simulink library "DiSC_ToolboxOpal_V12"  (R2012b)
settings: Solver=ode45  StartTime=0.0  StopTime=10.0  RelTol=1e-3
undefined symbols (not defined in the file or in its folder): SamplingTime
(part 2 of 5)

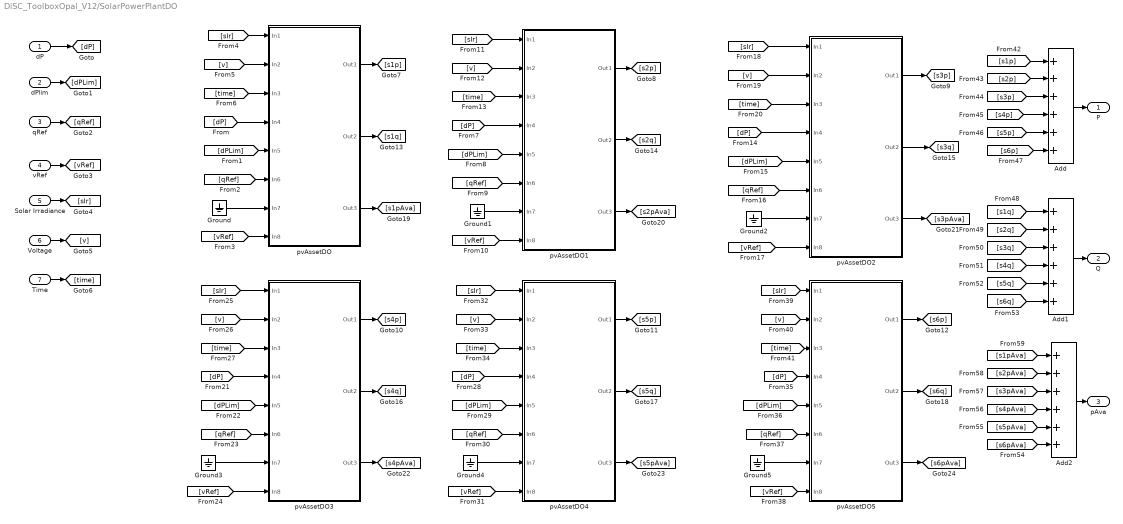
== system DiSC_ToolboxOpal_V12/SolarPowerPlantDO ==
  dP : Inport
  dPlim : Inport  Port=2
  qRef : Inport  Port=3
  vRef : Inport  Port=4
  Solar Irradiance : Inport  Port=5
  Voltage : Inport  Port=6
  Time : Inport  Port=7
  Add : Sum  Inputs=++++++
  Add1 : Sum  Inputs=++++++
  Add2 : Sum  Inputs=++++++
  Ground{,1..5} (6 alike) : Ground
  pvAssetDO : Subsystem
      mask help:
      | %pvAssetDO implements a simple P,Q controllable solar PV system using MATLAB embedded function.
      |     %   The pvAsset can be set to follow an active power reference, output
      |     %   maximum power available or derate power. It can also, at the same
      |     %   time be set to follow a reactive power reference, output the
      |     %   minimum reactive power according to the power factor or try to keep
      |     %   a voltage reference in the coupling point by controlling reactive
      |     %   power output.
      |     %
      |     %
      |     % Revision:
      |     % 19-06-2014, R. Pedersen, Aalborg University. Notes:
      |     % R. Pedersen 11-6-2014, Aalborg University
      |     % 29-11-2014, R. Olsen/M. Kemal, Aalborg University (Simulink)
      |     % 20-06-2015, F. Iov/M. Kemal, Aalborg University (Simulink toolbox for OPAL)
      |
      |                 % Input:
      |             %   - s [w/m^2], is the solar irradiance.
      |             %   - v [V], is the voltage at the connection point.
      |             %   - dP [PU], is the reference to active power change (curtailment).
      |             %   - dPlim [PU], is the reference to derated power (derate)
      |             %   - qRef [VAR], is the reactive power reference.
      |             %   - vRef [V], is the voltage reference.
      |             %
      |             % Output:
      |             %   - p [W], is the active power output
      |             %   - q [VAR], is the reactive power output
      |             %   - pAva [W], is the available power
      mask Help:
      | %pvAssetDO implements a simple P,Q controllable solar PV system using MATLAB embedded function.
      |     %   The pvAsset can be set to follow an active power reference, output
      |     %   maximum power available or derate power. It can also, at the same
      |     %   time be set to follow a reactive power reference, output the
      |     %   minimum reactive power according to the power factor or try to keep
      |     %   a voltage reference in the coupling point by controlling reactive
      |     %   power output.
      |     %
      |     %
      |     % Revision:
      |     % 19-06-2014, R. Pedersen, Aalborg University. Notes:
      |     % R. Pedersen 11-6-2014, Aalborg University
      |     % 29-11-2014, R. Olsen/M. Kemal, Aalborg University (Simulink)
      |     % 20-06-2015, F. Iov/M. Kemal, Aalborg University (Simulink toolbox for OPAL)
      | 
      |                 % Input:
      |             %   - s [w/m^2], is the solar irradiance.
      |             %   - v [V], is the voltage at the connection point.
      |             %   - dP [W], is the reference to active power change.
      |             %   - dPlim [W], is the reference to derated power.
      |             %   - qRef [VAR], is the reactive power reference.
      |             %   - vRef [V], is the voltage reference.
      |             %
      |             % Output:
      |             %   - p [W], is the active power output
      |             %   - q [VAR], is the reactive power output
      |             %   - pAva [W], is the available power
      mask Display:
      | %image(imread( 'PhotoVoltaic.png'))
      | port_label( 'output',1, 'p')
      | port_label( 'output',2, 'q')
      | port_label( 'output',3, 'pAva')
      | 
      | 
      | port_label( 'input',1, 'solarIrr')
      | port_label( 'input',2, 'vMeas')
      | port_label( 'input',3, 'time')
      | port_label( 'input',4, 'dp')
      | port_label( 'input',5, 'dplim')
      | port_label( 'input',6, 'qRef')
      | port_label( 'input',7, 'qMode')
      | port_label( 'input',8, 'vRef')
  pvAssetDO1 : Subsystem
      mask help:
      | %pvAssetDO implements a simple P,Q controllable solar PV system using MATLAB embedded function.
      |     %   The pvAsset can be set to follow an active power reference, output
      |     %   maximum power available or derate power. It can also, at the same
      |     %   time be set to follow a reactive power reference, output the
      |     %   minimum reactive power according to the power factor or try to keep
      |     %   a voltage reference in the coupling point by controlling reactive
      |     %   power output.
      |     %
      |     %
      |     % Revision:
      |     % 19-06-2014, R. Pedersen, Aalborg University. Notes:
      |     % R. Pedersen 11-6-2014, Aalborg University
      |     % 29-11-2014, R. Olsen/M. Kemal, Aalborg University (Simulink)
      |     % 20-06-2015, F. Iov/M. Kemal, Aalborg University (Simulink toolbox for OPAL)
      |
      |                 % Input:
      |             %   - s [w/m^2], is the solar irradiance.
      |             %   - v [V], is the voltage at the connection point.
      |             %   - dP [PU], is the reference to active power change (curtailment).
      |             %   - dPlim [PU], is the reference to derated power (derate)
      |             %   - qRef [VAR], is the reactive power reference.
      |             %   - vRef [V], is the voltage reference.
      |             %
      |             % Output:
      |             %   - p [W], is the active power output
      |             %   - q [VAR], is the reactive power output
      |             %   - pAva [W], is the available power
      mask Help:
      | %pvAssetDO implements a simple P,Q controllable solar PV system using MATLAB embedded function.
      |     %   The pvAsset can be set to follow an active power reference, output
      |     %   maximum power available or derate power. It can also, at the same
      |     %   time be set to follow a reactive power reference, output the
      |     %   minimum reactive power according to the power factor or try to keep
      |     %   a voltage reference in the coupling point by controlling reactive
      |     %   power output.
      |     %
      |     %
      |     % Revision:
      |     % 19-06-2014, R. Pedersen, Aalborg University. Notes:
      |     % R. Pedersen 11-6-2014, Aalborg University
      |     % 29-11-2014, R. Olsen/M. Kemal, Aalborg University (Simulink)
      |     % 20-06-2015, F. Iov/M. Kemal, Aalborg University (Simulink toolbox for OPAL)
      | 
      |                 % Input:
      |             %   - s [w/m^2], is the solar irradiance.
      |             %   - v [V], is the voltage at the connection point.
      |             %   - dP [W], is the reference to active power change.
      |             %   - dPlim [W], is the reference to derated power.
      |             %   - qRef [VAR], is the reactive power reference.
      |             %   - vRef [V], is the voltage reference.
      |             %
      |             % Output:
      |             %   - p [W], is the active power output
      |             %   - q [VAR], is the reactive power output
      |             %   - pAva [W], is the available power
      mask Display:
      | %image(imread( 'PhotoVoltaic.png'))
      | port_label( 'output',1, 'p')
      | port_label( 'output',2, 'q')
      | port_label( 'output',3, 'pAva')
      | 
      | 
      | port_label( 'input',1, 'solarIrr')
      | port_label( 'input',2, 'vMeas')
      | port_label( 'input',3, 'time')
      | port_label( 'input',4, 'dp')
      | port_label( 'input',5, 'dplim')
      | port_label( 'input',6, 'qRef')
      | port_label( 'input',7, 'qMode')
      | port_label( 'input',8, 'vRef')
  pvAssetDO2 : Subsystem
      mask help:
      | %pvAssetDO implements a simple P,Q controllable solar PV system using MATLAB embedded function.
      |     %   The pvAsset can be set to follow an active power reference, output
      |     %   maximum power available or derate power. It can also, at the same
      |     %   time be set to follow a reactive power reference, output the
      |     %   minimum reactive power according to the power factor or try to keep
      |     %   a voltage reference in the coupling point by controlling reactive
      |     %   power output.
      |     %
      |     %
      |     % Revision:
      |     % 19-06-2014, R. Pedersen, Aalborg University. Notes:
      |     % R. Pedersen 11-6-2014, Aalborg University
      |     % 29-11-2014, R. Olsen/M. Kemal, Aalborg University (Simulink)
      |     % 20-06-2015, F. Iov/M. Kemal, Aalborg University (Simulink toolbox for OPAL)
      |
      |                 % Input:
      |             %   - s [w/m^2], is the solar irradiance.
      |             %   - v [V], is the voltage at the connection point.
      |             %   - dP [PU], is the reference to active power change (curtailment).
      |             %   - dPlim [PU], is the reference to derated power (derate)
      |             %   - qRef [VAR], is the reactive power reference.
      |             %   - vRef [V], is the voltage reference.
      |             %
      |             % Output:
      |             %   - p [W], is the active power output
      |             %   - q [VAR], is the reactive power output
      |             %   - pAva [W], is the available power
      mask Help:
      | %pvAssetDO implements a simple P,Q controllable solar PV system using MATLAB embedded function.
      |     %   The pvAsset can be set to follow an active power reference, output
      |     %   maximum power available or derate power. It can also, at the same
      |     %   time be set to follow a reactive power reference, output the
      |     %   minimum reactive power according to the power factor or try to keep
      |     %   a voltage reference in the coupling point by controlling reactive
      |     %   power output.
      |     %
      |     %
      |     % Revision:
      |     % 19-06-2014, R. Pedersen, Aalborg University. Notes:
      |     % R. Pedersen 11-6-2014, Aalborg University
      |     % 29-11-2014, R. Olsen/M. Kemal, Aalborg University (Simulink)
      |     % 20-06-2015, F. Iov/M. Kemal, Aalborg University (Simulink toolbox for OPAL)
      | 
      |                 % Input:
      |             %   - s [w/m^2], is the solar irradiance.
      |             %   - v [V], is the voltage at the connection point.
      |             %   - dP [W], is the reference to active power change.
      |             %   - dPlim [W], is the reference to derated power.
      |             %   - qRef [VAR], is the reactive power reference.
      |             %   - vRef [V], is the voltage reference.
      |             %
      |             % Output:
      |             %   - p [W], is the active power output
      |             %   - q [VAR], is the reactive power output
      |             %   - pAva [W], is the available power
      mask Display:
      | %image(imread( 'PhotoVoltaic.png'))
      | port_label( 'output',1, 'p')
      | port_label( 'output',2, 'q')
      | port_label( 'output',3, 'pAva')
      | 
      | 
      | port_label( 'input',1, 'solarIrr')
      | port_label( 'input',2, 'vMeas')
      | port_label( 'input',3, 'time')
      | port_label( 'input',4, 'dp')
      | port_label( 'input',5, 'dplim')
      | port_label( 'input',6, 'qRef')
      | port_label( 'input',7, 'qMode')
      | port_label( 'input',8, 'vRef')
  pvAssetDO3 : Subsystem
      mask help:
      | %pvAssetDO implements a simple P,Q controllable solar PV system using MATLAB embedded function.
      |     %   The pvAsset can be set to follow an active power reference, output
      |     %   maximum power available or derate power. It can also, at the same
      |     %   time be set to follow a reactive power reference, output the
      |     %   minimum reactive power according to the power factor or try to keep
      |     %   a voltage reference in the coupling point by controlling reactive
      |     %   power output.
      |     %
      |     %
      |     % Revision:
      |     % 19-06-2014, R. Pedersen, Aalborg University. Notes:
      |     % R. Pedersen 11-6-2014, Aalborg University
      |     % 29-11-2014, R. Olsen/M. Kemal, Aalborg University (Simulink)
      |     % 20-06-2015, F. Iov/M. Kemal, Aalborg University (Simulink toolbox for OPAL)
      |
      |                 % Input:
      |             %   - s [w/m^2], is the solar irradiance.
      |             %   - v [V], is the voltage at the connection point.
      |             %   - dP [PU], is the reference to active power change (curtailment).
      |             %   - dPlim [PU], is the reference to derated power (derate)
      |             %   - qRef [VAR], is the reactive power reference.
      |             %   - vRef [V], is the voltage reference.
      |             %
      |             % Output:
      |             %   - p [W], is the active power output
      |             %   - q [VAR], is the reactive power output
      |             %   - pAva [W], is the available power
      mask Help:
      | %pvAssetDO implements a simple P,Q controllable solar PV system using MATLAB embedded function.
      |     %   The pvAsset can be set to follow an active power reference, output
      |     %   maximum power available or derate power. It can also, at the same
      |     %   time be set to follow a reactive power reference, output the
      |     %   minimum reactive power according to the power factor or try to keep
      |     %   a voltage reference in the coupling point by controlling reactive
      |     %   power output.
      |     %
      |     %
      |     % Revision:
      |     % 19-06-2014, R. Pedersen, Aalborg University. Notes:
      |     % R. Pedersen 11-6-2014, Aalborg University
      |     % 29-11-2014, R. Olsen/M. Kemal, Aalborg University (Simulink)
      |     % 20-06-2015, F. Iov/M. Kemal, Aalborg University (Simulink toolbox for OPAL)
      | 
      |                 % Input:
      |             %   - s [w/m^2], is the solar irradiance.
      |             %   - v [V], is the voltage at the connection point.
      |             %   - dP [W], is the reference to active power change.
      |             %   - dPlim [W], is the reference to derated power.
      |             %   - qRef [VAR], is the reactive power reference.
      |             %   - vRef [V], is the voltage reference.
      |             %
      |             % Output:
      |             %   - p [W], is the active power output
      |             %   - q [VAR], is the reactive power output
      |             %   - pAva [W], is the available power
      mask Display:
      | %image(imread( 'PhotoVoltaic.png'))
      | port_label( 'output',1, 'p')
      | port_label( 'output',2, 'q')
      | port_label( 'output',3, 'pAva')
      | 
      | 
      | port_label( 'input',1, 'solarIrr')
      | port_label( 'input',2, 'vMeas')
      | port_label( 'input',3, 'time')
      | port_label( 'input',4, 'dp')
      | port_label( 'input',5, 'dplim')
      | port_label( 'input',6, 'qRef')
      | port_label( 'input',7, 'qMode')
      | port_label( 'input',8, 'vRef')
  pvAssetDO4 : Subsystem
      mask help:
      | %pvAssetDO implements a simple P,Q controllable solar PV system using MATLAB embedded function.
      |     %   The pvAsset can be set to follow an active power reference, output
      |     %   maximum power available or derate power. It can also, at the same
      |     %   time be set to follow a reactive power reference, output the
      |     %   minimum reactive power according to the power factor or try to keep
      |     %   a voltage reference in the coupling point by controlling reactive
      |     %   power output.
      |     %
      |     %
      |     % Revision:
      |     % 19-06-2014, R. Pedersen, Aalborg University. Notes:
      |     % R. Pedersen 11-6-2014, Aalborg University
      |     % 29-11-2014, R. Olsen/M. Kemal, Aalborg University (Simulink)
      |     % 20-06-2015, F. Iov/M. Kemal, Aalborg University (Simulink toolbox for OPAL)
      |
      |                 % Input:
      |             %   - s [w/m^2], is the solar irradiance.
      |             %   - v [V], is the voltage at the connection point.
      |             %   - dP [PU], is the reference to active power change (curtailment).
      |             %   - dPlim [PU], is the reference to derated power (derate)
      |             %   - qRef [VAR], is the reactive power reference.
      |             %   - vRef [V], is the voltage reference.
      |             %
      |             % Output:
      |             %   - p [W], is the active power output
      |             %   - q [VAR], is the reactive power output
      |             %   - pAva [W], is the available power
      mask Help:
      | %pvAssetDO implements a simple P,Q controllable solar PV system using MATLAB embedded function.
      |     %   The pvAsset can be set to follow an active power reference, output
      |     %   maximum power available or derate power. It can also, at the same
      |     %   time be set to follow a reactive power reference, output the
      |     %   minimum reactive power according to the power factor or try to keep
      |     %   a voltage reference in the coupling point by controlling reactive
      |     %   power output.
      |     %
      |     %
      |     % Revision:
      |     % 19-06-2014, R. Pedersen, Aalborg University. Notes:
      |     % R. Pedersen 11-6-2014, Aalborg University
      |     % 29-11-2014, R. Olsen/M. Kemal, Aalborg University (Simulink)
      |     % 20-06-2015, F. Iov/M. Kemal, Aalborg University (Simulink toolbox for OPAL)
      | 
      |                 % Input:
      |             %   - s [w/m^2], is the solar irradiance.
      |             %   - v [V], is the voltage at the connection point.
      |             %   - dP [W], is the reference to active power change.
      |             %   - dPlim [W], is the reference to derated power.
      |             %   - qRef [VAR], is the reactive power reference.
      |             %   - vRef [V], is the voltage reference.
      |             %
      |             % Output:
      |             %   - p [W], is the active power output
      |             %   - q [VAR], is the reactive power output
      |             %   - pAva [W], is the available power
      mask Display:
      | %image(imread( 'PhotoVoltaic.png'))
      | port_label( 'output',1, 'p')
      | port_label( 'output',2, 'q')
      | port_label( 'output',3, 'pAva')
      | 
      | 
      | port_label( 'input',1, 'solarIrr')
      | port_label( 'input',2, 'vMeas')
      | port_label( 'input',3, 'time')
      | port_label( 'input',4, 'dp')
      | port_label( 'input',5, 'dplim')
      | port_label( 'input',6, 'qRef')
      | port_label( 'input',7, 'qMode')
      | port_label( 'input',8, 'vRef')
  pvAssetDO5 : Subsystem
      mask help:
      | %pvAssetDO implements a simple P,Q controllable solar PV system using MATLAB embedded function.
      |     %   The pvAsset can be set to follow an active power reference, output
      |     %   maximum power available or derate power. It can also, at the same
      |     %   time be set to follow a reactive power reference, output the
      |     %   minimum reactive power according to the power factor or try to keep
      |     %   a voltage reference in the coupling point by controlling reactive
      |     %   power output.
      |     %
      |     %
      |     % Revision:
      |     % 19-06-2014, R. Pedersen, Aalborg University. Notes:
      |     % R. Pedersen 11-6-2014, Aalborg University
      |     % 29-11-2014, R. Olsen/M. Kemal, Aalborg University (Simulink)
      |     % 20-06-2015, F. Iov/M. Kemal, Aalborg University (Simulink toolbox for OPAL)
      |
      |                 % Input:
      |             %   - s [w/m^2], is the solar irradiance.
      |             %   - v [V], is the voltage at the connection point.
      |             %   - dP [PU], is the reference to active power change (curtailment).
      |             %   - dPlim [PU], is the reference to derated power (derate)
      |             %   - qRef [VAR], is the reactive power reference.
      |             %   - vRef [V], is the voltage reference.
      |             %
      |             % Output:
      |             %   - p [W], is the active power output
      |             %   - q [VAR], is the reactive power output
      |             %   - pAva [W], is the available power
      mask Help:
      | %pvAssetDO implements a simple P,Q controllable solar PV system using MATLAB embedded function.
      |     %   The pvAsset can be set to follow an active power reference, output
      |     %   maximum power available or derate power. It can also, at the same
      |     %   time be set to follow a reactive power reference, output the
      |     %   minimum reactive power according to the power factor or try to keep
      |     %   a voltage reference in the coupling point by controlling reactive
      |     %   power output.
      |     %
      |     %
      |     % Revision:
      |     % 19-06-2014, R. Pedersen, Aalborg University. Notes:
      |     % R. Pedersen 11-6-2014, Aalborg University
      |     % 29-11-2014, R. Olsen/M. Kemal, Aalborg University (Simulink)
      |     % 20-06-2015, F. Iov/M. Kemal, Aalborg University (Simulink toolbox for OPAL)
      | 
      |                 % Input:
      |             %   - s [w/m^2], is the solar irradiance.
      |             %   - v [V], is the voltage at the connection point.
      |             %   - dP [W], is the reference to active power change.
      |             %   - dPlim [W], is the reference to derated power.
      |             %   - qRef [VAR], is the reactive power reference.
      |             %   - vRef [V], is the voltage reference.
      |             %
      |             % Output:
      |             %   - p [W], is the active power output
      |             %   - q [VAR], is the reactive power output
      |             %   - pAva [W], is the available power
      mask Display:
      | %image(imread( 'PhotoVoltaic.png'))
      | port_label( 'output',1, 'p')
      | port_label( 'output',2, 'q')
      | port_label( 'output',3, 'pAva')
      | 
      | 
      | port_label( 'input',1, 'solarIrr')
      | port_label( 'input',2, 'vMeas')
      | port_label( 'input',3, 'time')
      | port_label( 'input',4, 'dp')
      | port_label( 'input',5, 'dplim')
      | port_label( 'input',6, 'qRef')
      | port_label( 'input',7, 'qMode')
      | port_label( 'input',8, 'vRef')
  P : Outport
  Q : Outport  Port=2
  pAva : Outport  Port=3
  wires:
  [s1pAva] -> Add2/1
  [s2pAva] -> Add2/2
  [s3pAva] -> Add2/3
  [s4pAva] -> Add2/4
  [s5pAva] -> Add2/5
  [s6pAva] -> Add2/6
  pvAssetDO5/3(Out3) -> [s6pAva]
  pvAssetDO4/3(Out3) -> [s5pAva]
  pvAssetDO3/3(Out3) -> [s4pAva]
  pvAssetDO1/3(Out3) -> [s2pAva]
  pvAssetDO/3(Out3) -> [s1pAva]
  Add2/1 -> pAva/1
  [s6q] -> Add1/6
  [s5q] -> Add1/5
  [s4q] -> Add1/4
  [s3q] -> Add1/3
  [s2q] -> Add1/2
  [s1q] -> Add1/1
  Add1/1 -> Q/1
  pvAssetDO5/2(Out2) -> [s6q]
  pvAssetDO4/2(Out2) -> [s5q]
  pvAssetDO3/2(Out2) -> [s4q]
  pvAssetDO1/2(Out2) -> [s2q]
  pvAssetDO/2(Out2) -> [s1q]
  [s6p] -> Add/6
  [s5p] -> Add/5
  [s4p] -> Add/4
  [s3p] -> Add/3
  [s2p] -> Add/2
  [s1p] -> Add/1
  Add/1 -> P/1
  pvAssetDO5/1(Out1) -> [s6p]
  pvAssetDO4/1(Out1) -> [s5p]
  pvAssetDO3/1(Out1) -> [s4p]
  pvAssetDO1/1(Out1) -> [s2p]
  pvAssetDO/1(Out1) -> [s1p]
  [time] -> pvAssetDO5/3(In3)
  [v] -> pvAssetDO5/2(In2)
  [sIr] -> pvAssetDO5/1(In1)
  [vRef] -> pvAssetDO5/8(In8)
  [qRef] -> pvAssetDO5/6(In6)
  [dP] -> pvAssetDO5/4(In4)
  [dPLim] -> pvAssetDO5/5(In5)
  [time] -> pvAssetDO4/3(In3)
  [v] -> pvAssetDO4/2(In2)
  [sIr] -> pvAssetDO4/1(In1)
  [vRef] -> pvAssetDO4/8(In8)
  [qRef] -> pvAssetDO4/6(In6)
  [dP] -> pvAssetDO4/4(In4)
  [dPLim] -> pvAssetDO4/5(In5)
  [time] -> pvAssetDO3/3(In3)
  [v] -> pvAssetDO3/2(In2)
  [sIr] -> pvAssetDO3/1(In1)
  [vRef] -> pvAssetDO3/8(In8)
  [qRef] -> pvAssetDO3/6(In6)
  [dP] -> pvAssetDO3/4(In4)
  [dPLim] -> pvAssetDO3/5(In5)
  [time] -> pvAssetDO2/3(In3)
  [v] -> pvAssetDO2/2(In2)
  [sIr] -> pvAssetDO2/1(In1)
  [vRef] -> pvAssetDO2/8(In8)
  [qRef] -> pvAssetDO2/6(In6)
  [dP] -> pvAssetDO2/4(In4)
  [dPLim] -> pvAssetDO2/5(In5)
  [time] -> pvAssetDO1/3(In3)
  [v] -> pvAssetDO1/2(In2)
  [sIr] -> pvAssetDO1/1(In1)
  [qRef] -> pvAssetDO1/6(In6)
  [dP] -> pvAssetDO1/4(In4)
  [dPLim] -> pvAssetDO1/5(In5)
  [time] -> pvAssetDO/3(In3)
  Time/1 -> [time]
  [v] -> pvAssetDO/2(In2)
  Voltage/1 -> [v]
  [sIr] -> pvAssetDO/1(In1)
  Solar Irradiance/1 -> [sIr]
  [vRef] -> pvAssetDO/8(In8)
  vRef/1 -> [vRef]
  [qRef] -> pvAssetDO/6(In6)
  qRef/1 -> [qRef]
  [dP] -> pvAssetDO/4(In4)
  [dPLim] -> pvAssetDO/5(In5)
  dPlim/1 -> [dPLim]
  dP/1 -> [dP]
  [vRef] -> pvAssetDO1/8(In8)
  Ground/1 -> pvAssetDO/7(In7)
  Ground1/1 -> pvAssetDO1/7(In7)
  pvAssetDO2/1(Out1) -> [s3p]
  pvAssetDO2/2(Out2) -> [s3q]
  pvAssetDO2/3(Out3) -> [s3pAva]
  Ground2/1 -> pvAssetDO2/7(In7)
  Ground3/1 -> pvAssetDO3/7(In7)
  Ground4/1 -> pvAssetDO4/7(In7)
  Ground5/1 -> pvAssetDO5/7(In7)

== system DiSC_ToolboxOpal_V12/SuperMarket ==
  exeDefrost : Inport
  pRS : Inport  Port=2
  time : Inport  Port=3
  MATLAB Function : MATLAB Function  TreatAsAtomicUnit=on
  p : Outport
  q : Outport  Port=2
  timeReady : Outport  Port=3
  timeDefrost : Outport  Port=4
  wires:
  MATLAB Function/2(q) -> q/1
  MATLAB Function/3(timeReady) -> timeReady/1
  pRS/1 -> MATLAB Function/2(pRS)
  time/1 -> MATLAB Function/3(t)
  exeDefrost/1 -> MATLAB Function/1(exeDefrost)
  MATLAB Function/4(timeDefrost) -> timeDefrost/1
  MATLAB Function/1(p) -> p/1

== system DiSC_ToolboxOpal_V12/Tap Changer ==
  In1 : Inport
  In2 : Inport  Port=2
  In3 : Inport  Port=3
  In4 : Inport  Port=4
  In5 : Inport  Port=5
  In6 : Inport  Port=6
  MATLAB Function : MATLAB Function  TreatAsAtomicUnit=on
  Out1 : Outport
  Out2 : Outport  Port=2
  Out3 : Outport  Port=3
  wires:
  MATLAB Function/1(y1) -> Out1/1
  In3/1 -> MATLAB Function/3(uRef)
  In6/1 -> MATLAB Function/6(time)
  MATLAB Function/3(y3) -> Out2/1
  In4/1 -> MATLAB Function/4(mode)
  MATLAB Function/2(y2) -> Out3/1
  In2/1 -> MATLAB Function/2(vRef)
  In5/1 -> MATLAB Function/5(day)
  In1/1 -> MATLAB Function/1(vMeas)

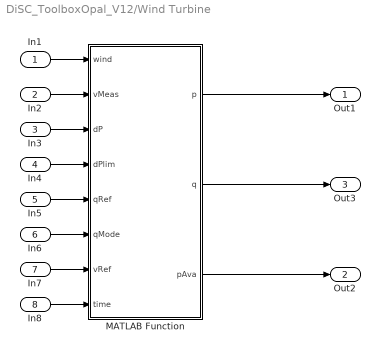
== system DiSC_ToolboxOpal_V12/Wind Turbine ==
  In1 : Inport
  In2 : Inport  Port=2
  In3 : Inport  Port=3
  In4 : Inport  Port=4
  In5 : Inport  Port=5
  In6 : Inport  Port=6
  In7 : Inport  Port=7
  In8 : Inport  Port=8
  MATLAB Function : MATLAB Function  TreatAsAtomicUnit=on
  Out1 : Outport
  Out2 : Outport  Port=2
  Out3 : Outport  Port=3
  wires:
  In8/1 -> MATLAB Function/8(time)
  In5/1 -> MATLAB Function/5(qRef)
  In6/1 -> MATLAB Function/6(qMode)
  In7/1 -> MATLAB Function/7(vRef)
  MATLAB Function/1(p) -> Out1/1
  In3/1 -> MATLAB Function/3(dP)
  In2/1 -> MATLAB Function/2(vMeas)
  MATLAB Function/2(q) -> Out3/1
  In4/1 -> MATLAB Function/4(dPlim)
  MATLAB Function/3(pAva) -> Out2/1
  In1/1 -> MATLAB Function/1(wind)

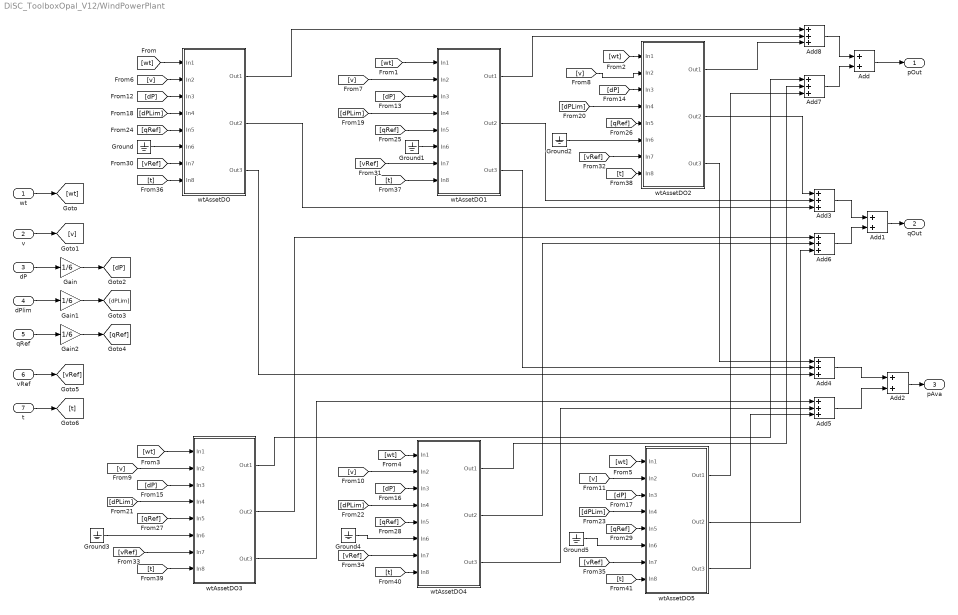
== system DiSC_ToolboxOpal_V12/WindPowerPlant ==
  wt : Inport
  v : Inport  Port=2
  dP : Inport  Port=3
  dPlim : Inport  Port=4
  qRef : Inport  Port=5
  vRef : Inport  Port=6
  t : Inport  Port=7
  Add : Sum
  Add1 : Sum
  Add2 : Sum
  Add{3..8} (6 alike) : Sum  Inputs=+++
  Gain : Gain  Gain=1/6
  Gain1 : Gain  Gain=1/6
  Gain2 : Gain  Gain=1/6
  Ground{,1..5} (6 alike) : Ground
  wtAssetDO : Subsystem
      mask help:
      | %wtAssetS implements a simple P,Q controllable wind turbine system for Simulink.
      |     % This model works for Simulink and requires generatedWindFiles to
      |     % have been executed before running the simulink model
      |     %
      |     %   The wtAsset can be set to follow an active power reference, output
      |     %   maximum power available or curtail power. It can also, at the same
      |     %   time be set to follow a reactive power reference, output the
      |     %   minimum reactive power according to the power factor or try to keep
      |     %   a voltage reference in the coupling point by controlling reactive
      |     %   power output.
      |     %
      |     %   The model is partly based on the book
      |     %   "Optimal Control of Wind Energy Systems 2008".
      |     %
      |     %
      |     % Revision:
      |     % 23-05-2014, C. E. Sloth and R. Pedersen, Aalborg University. Notes:
      |     % 29-11-2014, R. Olsen/M. Kemal, Aalborg University (Simulink)
      |     % 20-06-2015, F. Iov/M. Kemal, Aalborg University (Simulink toolbox for OPAL)
      |             % Input:
      |             %   - w [m/s], is the wind speed.
      |             %   - v [PU], is the voltage at the connection point.
      |             %   - dP [PU], is the reference to active power change (curtailment).
      |             %   - dPlim [PU], is the reference to derated power (derate).
      |             %   - qRef [PU], is the reactive power reference.
      |             %   - vRef [PU], is the voltage reference.
      |             %
      |             % Output:
      |             %   - p [W], is active power outpur.
      |             %   - q [VAR], is reactive power output.
      |             %   - pAva [W], is the available active power
      mask Help:
      | %wtAssetS implements a simple P,Q controllable wind turbine system for Simulink.
      |     % This model works for Simulink and requires generatedWindFiles to
      |     % have been executed before running the simulink model
      |     %
      |     %   The wtAsset can be set to follow an active power reference, output
      |     %   maximum power available or curtail power. It can also, at the same
      |     %   time be set to follow a reactive power reference, output the
      |     %   minimum reactive power according to the power factor or try to keep
      |     %   a voltage reference in the coupling point by controlling reactive
      |     %   power output.
      |     %
      |     %   The model is partly based on the book
      |     %   "Optimal Control of Wind Energy Systems 2008".
      |     %
      |     %
      |     % Revision:
      |     % 23-05-2014, C. E. Sloth and R. Pedersen, Aalborg University. Notes:
      |     % 29-11-2014, R. Olsen/M. Kemal, Aalborg University (Simulink)
      |     % 20-06-2015, F. Iov/M. Kemal, Aalborg University (Simulink toolbox for OPAL)
      |             % Input:
      |             %   - w [m/s], is the wind speed.
      |             %   - v [PU], is the voltage at the connection point.
      |             %   - dP [PU], is the reference to active power change (curtailment).
      |             %   - dPlim [PU], is the reference to derated power (derate).
      |             %   - qRef [PU], is the reactive power reference.
      |             %   - vRef [PU], is the voltage reference.
      |             %
      |             % Output:
      |             %   - p [W], is active power outpur.
      |             %   - q [VAR], is reactive power output.
      |             %   - pAva [W], is the available active power
      mask Display:
      | %image(imread( 'windTurbine.jpg'))
      | port_label( 'output',1, 'p')
      | port_label( 'output',2, 'q')
      | port_label( 'output',3, 'pAva')
      | 
      | 
      | port_label( 'input',1, 'wind')
      | port_label( 'input',2, 'vMeas')
      | port_label( 'input',3, 'dp')
      | port_label( 'input',4, 'dplim')
      | port_label( 'input',5, 'qRef')
      | port_label( 'input',6, 'qMode')
      | port_label( 'input',7, 'vRef')
      | port_label( 'input',8, 'time')
  wtAssetDO1 : Subsystem
      mask help:
      | %wtAssetS implements a simple P,Q controllable wind turbine system for Simulink.
      |     % This model works for Simulink and requires generatedWindFiles to
      |     % have been executed before running the simulink model
      |     %
      |     %   The wtAsset can be set to follow an active power reference, output
      |     %   maximum power available or curtail power. It can also, at the same
      |     %   time be set to follow a reactive power reference, output the
      |     %   minimum reactive power according to the power factor or try to keep
      |     %   a voltage reference in the coupling point by controlling reactive
      |     %   power output.
      |     %
      |     %   The model is partly based on the book
      |     %   "Optimal Control of Wind Energy Systems 2008".
      |     %
      |     %
      |     % Revision:
      |     % 23-05-2014, C. E. Sloth and R. Pedersen, Aalborg University. Notes:
      |     % 29-11-2014, R. Olsen/M. Kemal, Aalborg University (Simulink)
      |     % 20-06-2015, F. Iov/M. Kemal, Aalborg University (Simulink toolbox for OPAL)
      |             % Input:
      |             %   - w [m/s], is the wind speed.
      |             %   - v [PU], is the voltage at the connection point.
      |             %   - dP [PU], is the reference to active power change (curtailment).
      |             %   - dPlim [PU], is the reference to derated power (derate).
      |             %   - qRef [PU], is the reactive power reference.
      |             %   - vRef [PU], is the voltage reference.
      |             %
      |             % Output:
      |             %   - p [W], is active power outpur.
      |             %   - q [VAR], is reactive power output.
      |             %   - pAva [W], is the available active power
      mask Help:
      | %wtAssetS implements a simple P,Q controllable wind turbine system for Simulink.
      |     % This model works for Simulink and requires generatedWindFiles to
      |     % have been executed before running the simulink model
      |     %
      |     %   The wtAsset can be set to follow an active power reference, output
      |     %   maximum power available or curtail power. It can also, at the same
      |     %   time be set to follow a reactive power reference, output the
      |     %   minimum reactive power according to the power factor or try to keep
      |     %   a voltage reference in the coupling point by controlling reactive
      |     %   power output.
      |     %
      |     %   The model is partly based on the book
      |     %   "Optimal Control of Wind Energy Systems 2008".
      |     %
      |     %
      |     % Revision:
      |     % 23-05-2014, C. E. Sloth and R. Pedersen, Aalborg University. Notes:
      |     % 29-11-2014, R. Olsen/M. Kemal, Aalborg University (Simulink)
      |     % 20-06-2015, F. Iov/M. Kemal, Aalborg University (Simulink toolbox for OPAL)
      |             % Input:
      |             %   - w [m/s], is the wind speed.
      |             %   - v [PU], is the voltage at the connection point.
      |             %   - dP [PU], is the reference to active power change (curtailment).
      |             %   - dPlim [PU], is the reference to derated power (derate).
      |             %   - qRef [PU], is the reactive power reference.
      |             %   - vRef [PU], is the voltage reference.
      |             %
      |             % Output:
      |             %   - p [W], is active power outpur.
      |             %   - q [VAR], is reactive power output.
      |             %   - pAva [W], is the available active power
      mask Display:
      | %image(imread( 'windTurbine.jpg'))
      | port_label( 'output',1, 'p')
      | port_label( 'output',2, 'q')
      | port_label( 'output',3, 'pAva')
      | 
      | 
      | port_label( 'input',1, 'wind')
      | port_label( 'input',2, 'vMeas')
      | port_label( 'input',3, 'dp')
      | port_label( 'input',4, 'dplim')
      | port_label( 'input',5, 'qRef')
      | port_label( 'input',6, 'qMode')
      | port_label( 'input',7, 'vRef')
      | port_label( 'input',8, 'time')
  wtAssetDO2 : Subsystem
      mask help:
      | %wtAssetS implements a simple P,Q controllable wind turbine system for Simulink.
      |     % This model works for Simulink and requires generatedWindFiles to
      |     % have been executed before running the simulink model
      |     %
      |     %   The wtAsset can be set to follow an active power reference, output
      |     %   maximum power available or curtail power. It can also, at the same
      |     %   time be set to follow a reactive power reference, output the
      |     %   minimum reactive power according to the power factor or try to keep
      |     %   a voltage reference in the coupling point by controlling reactive
      |     %   power output.
      |     %
      |     %   The model is partly based on the book
      |     %   "Optimal Control of Wind Energy Systems 2008".
      |     %
      |     %
      |     % Revision:
      |     % 23-05-2014, C. E. Sloth and R. Pedersen, Aalborg University. Notes:
      |     % 29-11-2014, R. Olsen/M. Kemal, Aalborg University (Simulink)
      |     % 20-06-2015, F. Iov/M. Kemal, Aalborg University (Simulink toolbox for OPAL)
      |             % Input:
      |             %   - w [m/s], is the wind speed.
      |             %   - v [PU], is the voltage at the connection point.
      |             %   - dP [PU], is the reference to active power change (curtailment).
      |             %   - dPlim [PU], is the reference to derated power (derate).
      |             %   - qRef [PU], is the reactive power reference.
      |             %   - vRef [PU], is the voltage reference.
      |             %
      |             % Output:
      |             %   - p [W], is active power outpur.
      |             %   - q [VAR], is reactive power output.
      |             %   - pAva [W], is the available active power
      mask Help:
      | %wtAssetS implements a simple P,Q controllable wind turbine system for Simulink.
      |     % This model works for Simulink and requires generatedWindFiles to
      |     % have been executed before running the simulink model
      |     %
      |     %   The wtAsset can be set to follow an active power reference, output
      |     %   maximum power available or curtail power. It can also, at the same
      |     %   time be set to follow a reactive power reference, output the
      |     %   minimum reactive power according to the power factor or try to keep
      |     %   a voltage reference in the coupling point by controlling reactive
      |     %   power output.
      |     %
      |     %   The model is partly based on the book
      |     %   "Optimal Control of Wind Energy Systems 2008".
      |     %
      |     %
      |     % Revision:
      |     % 23-05-2014, C. E. Sloth and R. Pedersen, Aalborg University. Notes:
      |     % 29-11-2014, R. Olsen/M. Kemal, Aalborg University (Simulink)
      |     % 20-06-2015, F. Iov/M. Kemal, Aalborg University (Simulink toolbox for OPAL)
      |             % Input:
      |             %   - w [m/s], is the wind speed.
      |             %   - v [PU], is the voltage at the connection point.
      |             %   - dP [PU], is the reference to active power change (curtailment).
      |             %   - dPlim [PU], is the reference to derated power (derate).
      |             %   - qRef [PU], is the reactive power reference.
      |             %   - vRef [PU], is the voltage reference.
      |             %
      |             % Output:
      |             %   - p [W], is active power outpur.
      |             %   - q [VAR], is reactive power output.
      |             %   - pAva [W], is the available active power
      mask Display:
      | %image(imread( 'windTurbine.jpg'))
      | port_label( 'output',1, 'p')
      | port_label( 'output',2, 'q')
      | port_label( 'output',3, 'pAva')
      | 
      | 
      | port_label( 'input',1, 'wind')
      | port_label( 'input',2, 'vMeas')
      | port_label( 'input',3, 'dp')
      | port_label( 'input',4, 'dplim')
      | port_label( 'input',5, 'qRef')
      | port_label( 'input',6, 'qMode')
      | port_label( 'input',7, 'vRef')
      | port_label( 'input',8, 'time')
  wtAssetDO3 : Subsystem
      mask help:
      | %wtAssetS implements a simple P,Q controllable wind turbine system for Simulink.
      |     % This model works for Simulink and requires generatedWindFiles to
      |     % have been executed before running the simulink model
      |     %
      |     %   The wtAsset can be set to follow an active power reference, output
      |     %   maximum power available or curtail power. It can also, at the same
      |     %   time be set to follow a reactive power reference, output the
      |     %   minimum reactive power according to the power factor or try to keep
      |     %   a voltage reference in the coupling point by controlling reactive
      |     %   power output.
      |     %
      |     %   The model is partly based on the book
      |     %   "Optimal Control of Wind Energy Systems 2008".
      |     %
      |     %
      |     % Revision:
      |     % 23-05-2014, C. E. Sloth and R. Pedersen, Aalborg University. Notes:
      |     % 29-11-2014, R. Olsen/M. Kemal, Aalborg University (Simulink)
      |     % 20-06-2015, F. Iov/M. Kemal, Aalborg University (Simulink toolbox for OPAL)
      |             % Input:
      |             %   - w [m/s], is the wind speed.
      |             %   - v [PU], is the voltage at the connection point.
      |             %   - dP [PU], is the reference to active power change (curtailment).
      |             %   - dPlim [PU], is the reference to derated power (derate).
      |             %   - qRef [PU], is the reactive power reference.
      |             %   - vRef [PU], is the voltage reference.
      |             %
      |             % Output:
      |             %   - p [W], is active power outpur.
      |             %   - q [VAR], is reactive power output.
      |             %   - pAva [W], is the available active power
      mask Help:
      | %wtAssetS implements a simple P,Q controllable wind turbine system for Simulink.
      |     % This model works for Simulink and requires generatedWindFiles to
      |     % have been executed before running the simulink model
      |     %
      |     %   The wtAsset can be set to follow an active power reference, output
      |     %   maximum power available or curtail power. It can also, at the same
      |     %   time be set to follow a reactive power reference, output the
      |     %   minimum reactive power according to the power factor or try to keep
      |     %   a voltage reference in the coupling point by controlling reactive
      |     %   power output.
      |     %
      |     %   The model is partly based on the book
      |     %   "Optimal Control of Wind Energy Systems 2008".
      |     %
      |     %
      |     % Revision:
      |     % 23-05-2014, C. E. Sloth and R. Pedersen, Aalborg University. Notes:
      |     % 29-11-2014, R. Olsen/M. Kemal, Aalborg University (Simulink)
      |     % 20-06-2015, F. Iov/M. Kemal, Aalborg University (Simulink toolbox for OPAL)
      |             % Input:
      |             %   - w [m/s], is the wind speed.
      |             %   - v [PU], is the voltage at the connection point.
      |             %   - dP [PU], is the reference to active power change (curtailment).
      |             %   - dPlim [PU], is the reference to derated power (derate).
      |             %   - qRef [PU], is the reactive power reference.
      |             %   - vRef [PU], is the voltage reference.
      |             %
      |             % Output:
      |             %   - p [W], is active power outpur.
      |             %   - q [VAR], is reactive power output.
      |             %   - pAva [W], is the available active power
      mask Display:
      | %image(imread( 'windTurbine.jpg'))
      | port_label( 'output',1, 'p')
      | port_label( 'output',2, 'q')
      | port_label( 'output',3, 'pAva')
      | 
      | 
      | port_label( 'input',1, 'wind')
      | port_label( 'input',2, 'vMeas')
      | port_label( 'input',3, 'dp')
      | port_label( 'input',4, 'dplim')
      | port_label( 'input',5, 'qRef')
      | port_label( 'input',6, 'qMode')
      | port_label( 'input',7, 'vRef')
      | port_label( 'input',8, 'time')
  wtAssetDO4 : Subsystem
      mask help:
      | %wtAssetS implements a simple P,Q controllable wind turbine system for Simulink.
      |     % This model works for Simulink and requires generatedWindFiles to
      |     % have been executed before running the simulink model
      |     %
      |     %   The wtAsset can be set to follow an active power reference, output
      |     %   maximum power available or curtail power. It can also, at the same
      |     %   time be set to follow a reactive power reference, output the
      |     %   minimum reactive power according to the power factor or try to keep
      |     %   a voltage reference in the coupling point by controlling reactive
      |     %   power output.
      |     %
      |     %   The model is partly based on the book
      |     %   "Optimal Control of Wind Energy Systems 2008".
      |     %
      |     %
      |     % Revision:
      |     % 23-05-2014, C. E. Sloth and R. Pedersen, Aalborg University. Notes:
      |     % 29-11-2014, R. Olsen/M. Kemal, Aalborg University (Simulink)
      |     % 20-06-2015, F. Iov/M. Kemal, Aalborg University (Simulink toolbox for OPAL)
      |             % Input:
      |             %   - w [m/s], is the wind speed.
      |             %   - v [PU], is the voltage at the connection point.
      |             %   - dP [PU], is the reference to active power change (curtailment).
      |             %   - dPlim [PU], is the reference to derated power (derate).
      |             %   - qRef [PU], is the reactive power reference.
      |             %   - vRef [PU], is the voltage reference.
      |             %
      |             % Output:
      |             %   - p [W], is active power outpur.
      |             %   - q [VAR], is reactive power output.
      |             %   - pAva [W], is the available active power
      mask Help:
      | %wtAssetS implements a simple P,Q controllable wind turbine system for Simulink.
      |     % This model works for Simulink and requires generatedWindFiles to
      |     % have been executed before running the simulink model
      |     %
      |     %   The wtAsset can be set to follow an active power reference, output
      |     %   maximum power available or curtail power. It can also, at the same
      |     %   time be set to follow a reactive power reference, output the
      |     %   minimum reactive power according to the power factor or try to keep
      |     %   a voltage reference in the coupling point by controlling reactive
      |     %   power output.
      |     %
      |     %   The model is partly based on the book
      |     %   "Optimal Control of Wind Energy Systems 2008".
      |     %
      |     %
      |     % Revision:
      |     % 23-05-2014, C. E. Sloth and R. Pedersen, Aalborg University. Notes:
      |     % 29-11-2014, R. Olsen/M. Kemal, Aalborg University (Simulink)
      |     % 20-06-2015, F. Iov/M. Kemal, Aalborg University (Simulink toolbox for OPAL)
      |             % Input:
      |             %   - w [m/s], is the wind speed.
      |             %   - v [PU], is the voltage at the connection point.
      |             %   - dP [PU], is the reference to active power change (curtailment).
      |             %   - dPlim [PU], is the reference to derated power (derate).
      |             %   - qRef [PU], is the reactive power reference.
      |             %   - vRef [PU], is the voltage reference.
      |             %
      |             % Output:
      |             %   - p [W], is active power outpur.
      |             %   - q [VAR], is reactive power output.
      |             %   - pAva [W], is the available active power
      mask Display:
      | %image(imread( 'windTurbine.jpg'))
      | port_label( 'output',1, 'p')
      | port_label( 'output',2, 'q')
      | port_label( 'output',3, 'pAva')
      | 
      | 
      | port_label( 'input',1, 'wind')
      | port_label( 'input',2, 'vMeas')
      | port_label( 'input',3, 'dp')
      | port_label( 'input',4, 'dplim')
      | port_label( 'input',5, 'qRef')
      | port_label( 'input',6, 'qMode')
      | port_label( 'input',7, 'vRef')
      | port_label( 'input',8, 'time')
  wtAssetDO5 : Subsystem
      mask help:
      | %wtAssetS implements a simple P,Q controllable wind turbine system for Simulink.
      |     % This model works for Simulink and requires generatedWindFiles to
      |     % have been executed before running the simulink model
      |     %
      |     %   The wtAsset can be set to follow an active power reference, output
      |     %   maximum power available or curtail power. It can also, at the same
      |     %   time be set to follow a reactive power reference, output the
      |     %   minimum reactive power according to the power factor or try to keep
      |     %   a voltage reference in the coupling point by controlling reactive
      |     %   power output.
      |     %
      |     %   The model is partly based on the book
      |     %   "Optimal Control of Wind Energy Systems 2008".
      |     %
      |     %
      |     % Revision:
      |     % 23-05-2014, C. E. Sloth and R. Pedersen, Aalborg University. Notes:
      |     % 29-11-2014, R. Olsen/M. Kemal, Aalborg University (Simulink)
      |     % 20-06-2015, F. Iov/M. Kemal, Aalborg University (Simulink toolbox for OPAL)
      |             % Input:
      |             %   - w [m/s], is the wind speed.
      |             %   - v [PU], is the voltage at the connection point.
      |             %   - dP [PU], is the reference to active power change (curtailment).
      |             %   - dPlim [PU], is the reference to derated power (derate).
      |             %   - qRef [PU], is the reactive power reference.
      |             %   - vRef [PU], is the voltage reference.
      |             %
      |             % Output:
      |             %   - p [W], is active power outpur.
      |             %   - q [VAR], is reactive power output.
      |             %   - pAva [W], is the available active power
      mask Help:
      | %wtAssetS implements a simple P,Q controllable wind turbine system for Simulink.
      |     % This model works for Simulink and requires generatedWindFiles to
      |     % have been executed before running the simulink model
      |     %
      |     %   The wtAsset can be set to follow an active power reference, output
      |     %   maximum power available or curtail power. It can also, at the same
      |     %   time be set to follow a reactive power reference, output the
      |     %   minimum reactive power according to the power factor or try to keep
      |     %   a voltage reference in the coupling point by controlling reactive
      |     %   power output.
      |     %
      |     %   The model is partly based on the book
      |     %   "Optimal Control of Wind Energy Systems 2008".
      |     %
      |     %
      |     % Revision:
      |     % 23-05-2014, C. E. Sloth and R. Pedersen, Aalborg University. Notes:
      |     % 29-11-2014, R. Olsen/M. Kemal, Aalborg University (Simulink)
      |     % 20-06-2015, F. Iov/M. Kemal, Aalborg University (Simulink toolbox for OPAL)
      |             % Input:
      |             %   - w [m/s], is the wind speed.
      |             %   - v [PU], is the voltage at the connection point.
      |             %   - dP [PU], is the reference to active power change (curtailment).
      |             %   - dPlim [PU], is the reference to derated power (derate).
      |             %   - qRef [PU], is the reactive power reference.
      |             %   - vRef [PU], is the voltage reference.
      |             %
      |             % Output:
      |             %   - p [W], is active power outpur.
      |             %   - q [VAR], is reactive power output.
      |             %   - pAva [W], is the available active power
      mask Display:
      | %image(imread( 'windTurbine.jpg'))
      | port_label( 'output',1, 'p')
      | port_label( 'output',2, 'q')
      | port_label( 'output',3, 'pAva')
      | 
      | 
      | port_label( 'input',1, 'wind')
      | port_label( 'input',2, 'vMeas')
      | port_label( 'input',3, 'dp')
      | port_label( 'input',4, 'dplim')
      | port_label( 'input',5, 'qRef')
      | port_label( 'input',6, 'qMode')
      | port_label( 'input',7, 'vRef')
      | port_label( 'input',8, 'time')
  pOut : Outport
  qOut : Outport  Port=2
  pAva : Outport  Port=3
  wires:
  dP/1 -> Gain/1
  dPlim/1 -> Gain1/1
  qRef/1 -> Gain2/1
  wt/1 -> [wt]
  v/1 -> [v]
  Gain/1 -> [dP]
  Gain1/1 -> [dPLim]
  Gain2/1 -> [qRef]
  vRef/1 -> [vRef]
  t/1 -> [t]
  wtAssetDO2/1(Out1) -> Add8/3
  wtAssetDO1/1(Out1) -> Add8/2
  wtAssetDO/1(Out1) -> Add8/1
  wtAssetDO2/2(Out2) -> Add3/1
  wtAssetDO1/2(Out2) -> Add3/2
  wtAssetDO/2(Out2) -> Add3/3
  [wt] -> wtAssetDO/1(In1)
  [wt] -> wtAssetDO1/1(In1)
  [wt] -> wtAssetDO2/1(In1)
  [wt] -> wtAssetDO3/1(In1)
  [wt] -> wtAssetDO4/1(In1)
  [wt] -> wtAssetDO5/1(In1)
  [v] -> wtAssetDO/2(In2)
  [v] -> wtAssetDO1/2(In2)
  [v] -> wtAssetDO2/2(In2)
  [v] -> wtAssetDO3/2(In2)
  [v] -> wtAssetDO4/2(In2)
  [v] -> wtAssetDO5/2(In2)
  [dP] -> wtAssetDO/3(In3)
  [dP] -> wtAssetDO1/3(In3)
  [dP] -> wtAssetDO2/3(In3)
  [dP] -> wtAssetDO3/3(In3)
  [dP] -> wtAssetDO4/3(In3)
  [dP] -> wtAssetDO5/3(In3)
  [dPLim] -> wtAssetDO/4(In4)
  [dPLim] -> wtAssetDO1/4(In4)
  [dPLim] -> wtAssetDO2/4(In4)
  [dPLim] -> wtAssetDO3/4(In4)
  [dPLim] -> wtAssetDO4/4(In4)
  [dPLim] -> wtAssetDO5/4(In4)
  [qRef] -> wtAssetDO/5(In5)
  [qRef] -> wtAssetDO1/5(In5)
  [qRef] -> wtAssetDO2/5(In5)
  [qRef] -> wtAssetDO3/5(In5)
  [qRef] -> wtAssetDO4/5(In5)
  [qRef] -> wtAssetDO5/5(In5)
  [vRef] -> wtAssetDO1/7(In7)
  [vRef] -> wtAssetDO2/7(In7)
  [vRef] -> wtAssetDO3/7(In7)
  [vRef] -> wtAssetDO4/7(In7)
  [t] -> wtAssetDO/8(In8)
  [t] -> wtAssetDO1/8(In8)
  [t] -> wtAssetDO2/8(In8)
  [t] -> wtAssetDO3/8(In8)
  [t] -> wtAssetDO4/8(In8)
  wtAssetDO2/3(Out3) -> Add4/1
  wtAssetDO1/3(Out3) -> Add4/2
  wtAssetDO/3(Out3) -> Add4/3
  wtAssetDO5/3(Out3) -> Add5/3
  wtAssetDO4/3(Out3) -> Add5/2
  wtAssetDO3/3(Out3) -> Add5/1
  Add4/1 -> Add2/1
  Add5/1 -> Add2/2
  Add2/1 -> pAva/1
  wtAssetDO5/2(Out2) -> Add6/3
  wtAssetDO4/2(Out2) -> Add6/2
  wtAssetDO3/2(Out2) -> Add6/1
  Add3/1 -> Add1/1
  Add6/1 -> Add1/2
  Add1/1 -> qOut/1
  wtAssetDO5/1(Out1) -> Add7/3
  wtAssetDO4/1(Out1) -> Add7/2
  wtAssetDO3/1(Out1) -> Add7/1
  Add8/1 -> Add/1
  Add7/1 -> Add/2
  Add/1 -> pOut/1
  [vRef] -> wtAssetDO/7(In7)
  [t] -> wtAssetDO5/8(In8)
  [vRef] -> wtAssetDO5/7(In7)
  Ground/1 -> wtAssetDO/6(In6)
  Ground1/1 -> wtAssetDO1/6(In6)
  Ground2/1 -> wtAssetDO2/6(In6)
  Ground3/1 -> wtAssetDO3/6(In6)
  Ground4/1 -> wtAssetDO4/6(In6)
  Ground5/1 -> wtAssetDO5/6(In6)
